simulink library "DSP_FPGA_Accelerated_Toolbox"  (R2019b)
settings: Solver=VariableStepAuto  StartTime=0.0  StopTime=10.0  RelTol=1e-3
undefined symbols (not defined in the file or in its folder): a, b, c
libraries: hdlsllib x72, simulink x19, $bdroot x2
(part 1 of 3)
settings Model: Creator=E. Bailey Galacci  LastModifiedBy=Balad
settings SFSimCC: CustomCodeUndefinedFunction=UseInterfaceOnly

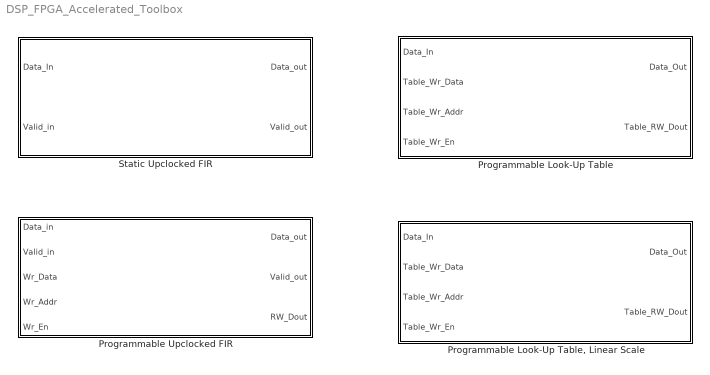
== system DSP_FPGA_Accelerated_Toolbox ==
  Programmable Look-Up Table : Subsystem  mask(Programmable Look-Up Table){TableFn=X_in.^0.5, maxInput=1, floor_in_tab=2^-15, error_cap_tab=.1, ERR_DIAG=off, N_bits_tab=4, M_bits_tab=5, igotthis=off, W_bits=32, F_bits=28, Table_Init=0, d=0}
      mask prompts: TableFn "Table Represented Function"; maxInput "Maximum Input Value"; floor_in_tab "Minimum Input Threshold"; error_cap_tab "Maximum Allowed Error (%)"; ERR_DIAG "Show Error Calculation"; N_bits_tab "N_bits"; M_bits_tab "M_bits"; igotthis "Manual Bit Definition Override"; W_bits "Word Bits"; F_bits "Fractional Bits"
      mask help:
      | A hardware-oriented implementation of a lookup table.
      | Provides a fairly resource efficient way to avoid hardware-difficult operations, such as logarithms or square roots.
      | Tables can be initialized on system startup and rewritten during runtime using the Table_Wr lines.
      | Min input cannot be 0, because inputs are pseudo-logarithmically spaced.
      mask init:
      | % things to display: table size, floor input?, max input, accuracy
      | % things to figure out: M_bits, N_bits, Min_val, X_in table, Y_out table,
      | % max_error, ram_size, table_size 
      | 
      | d = ceil(log2(maxInput));
      | if(igotthis)
      |     N_bits = N_bits_tab;
      |     M_bits = M_bits_tab;
      | else
      |     N_bits = ceil(log2(d-log2(floor_in_tab)+1));
      |     % M_bits needs to be defined later, as it must be just enough to meet
      |     % accuracy standards defined by user, with linear interpolation
      |     M_bits = 1; %this will be updated later as needed
      | end;
      | 
      | repeatFlag = true;
      | while(repeatFlag)
      |     % Define a N point log2 spaced range of inputs, from 2^(d-(2^N_bits -1)) to almost 2^(d+1), 
      |     % this effectively covers the user defined input range, down to a floor
      |     % value.
      |     X_in = zeros(1, 2^(M_bits+N_bits));
      |     addr = 1;
      |     for NShifts = 2^N_bits-1:-1:0
      |         for M = 0:2^M_bits - 1
      |             X_in(addr) = 2^(d-NShifts) + M*2^(d-NShifts-M_bits);
      |             addr = addr+1;
      |         end
      |     end
      | 
      |     % use function to define output. note: function must contain input X_in
      |     % within the string to work properly, and the only output of the function
      |     % must be Y_out.
      |     Y_out = eval(TableFn);
      | 
      |     ram_size = N_bits+M_bits;
      |     Table_Init = Y_out;
      |     figure(2); plot(X_in,Y_out, 'k*'); title('Table Initialized Function');
      |     max_val = 2^d+ (2^M_bits -1)*2^(d-M_bits);
      |     min_val = 2^(d-(2^N_bits-1));
      |     %set_param(gcb,'MaskDisplay',"disp(sprintf('Programmable Look-up Table\nMemory Used = %d samples and coeffs\nClock Rate Needed = %d Hz', FIR_Uprate*2, Max_Rate)); port_label('input',1,'data'); port_label('input',2,'valid'); port_label('input',3,'Wr_Data'); port_label('input',4,'Wr_Addr'); port_label('input',5,'Wr_En'); port_label('output',1,'data'); port_label('output',2,'valid'); port_label('output',3,'RW_Dout');")
      | 
      |     %%%%%%%%%% check and identify error %%%%%%%%%%%
      |     % Make some values for an "ideal" lookup table with log spaced points
      |     X_in_Ideal = logspace(log10(min_val), log10(max_val), 2^(ram_size+2));
      |     X_temp = X_in;
      |     X_in = X_in_Ideal;
      |     % identify the values of the function at X_in_Ideal
      |     Y_out_Ideal = eval(TableFn);
      | 
      |     % Get values for lookup table (already have X_in)
      |     X_in = X_temp;
      | 
      |     % Find lookup addresses for each point in X_in_Ideal
      |     x_addr = zeros(1,length(X_in_Ideal));
      |     for it = 1:length(X_in_Ideal)
      |         x_addr(it) = 2^ram_size;
      |         X_Shift = X_in_Ideal(it);
      |         while(X_Shift < X_in(x_addr(it)) && x_addr(it) ~= 1)
      |             x_addr(it) = x_addr(it) - 1;
      |         end
      |         if(x_addr(it)==0)
      |             x_addr(it) = 1;
      |         end
      |     end
      | 
      |     % Check for any possible out of bounds errors (handled similarly in
      |     % hardware)
      |     x_addr(x_addr == 2^ram_size) = 2^ram_size -1;
      | 
      |     % Get values for linear interpolation of X_in_Ideal
      |     x_low  = X_in(x_addr);
      |     x_high = X_in(x_addr+1);
      | 
      | 
      |     y_low  = Y_out(x_addr);
      |     y_high = Y_out(x_addr+1);
      |     slope  = (y_high-y_low) ./ (x_high - x_low);
      |     y_inter = slope.*(X_in_Ideal-x_low)+y_low;
      |     % percent error: obt-exp / exp
      |     %errorFloor = (Y_out_Ideal-y_low)./Y_out_Ideal;
      |     errorInter = (Y_out_Ideal-y_inter)./Y_out_Ideal;
      |     %maxFloorErr(ix) = 100*max(abs(errorFloor(ix, 2870:9839)));
      |     %maxInterErr(ix) = 100*max(abs(errorInter(ix, 2870:9839)));
      |     maxErr = max(abs(errorInter));
      |     
      |     %check while loop condition
      |     if(igotthis) 
      |         repeatFlag = false;
      |     else
      |         if(maxErr <= .01*error_cap_tab)
      |             repeatFlag = false;
      |             if(ERR_DIAG)
      |                 figure(1); 
      |                 subplot(2,1,1); semilogx(X_in_Ideal,y_inter, X_in_Ideal,Y_out_Ideal,X_in,Y_out,'k*'); title('Output Values over Input Range'); xlabel('Inputs'); ylabel('Outputs'); legend('Interpolated','Ideal','Table Points');
      |                 subplot(2,1,2); semilogx(X_in_Ideal,100*errorInter); title('Error of Output over Input Range'); xlabel('Inputs'); ylabel('Percent Error');
      |             end
      |         else
      |             if(ERR_DIAG)
      |                 f = msgbox(sprintf('Err = %.2d, M_bits = %d', maxErr, M_bits),'Configuring PLUT','replace');
      |             end
      |             if(maxErr > 8*.01*error_cap_tab)
      |                 M_bits = M_bits+3;
      |             elseif(maxErr > 4*.01*error_cap_tab)
      |                 M_bits = M_bits+2;
      |             else
      |                 M_bits = M_bits+1;
      |             end
      |         end
      |     end
      | end%end while loop
      | 
      | %maxFloorErrTot = max(maxFloorErr);
      | %maxInterErrTot = max(maxInterErr);
      | % things to display: table size, floor input?, max input, accuracy
      | 
      | set_param(gcb,'MaskDisplay',"disp(sprintf('Programmable Look-Up Table\nMemory Used = %d fixed point numbers\nInput Bounds: %.2d <= x <= %.2d\n Maximum Error: %.2d %', 2*2^ram_size, min_val, max_val, 100*maxErr)); port_label('input',1,'Data_In'); port_label('input',2,'Table_Wr_Data'); port_label('input',3,'Table_Wr_Addr'); port_label('input',4,'Table_Wr_En'); port_label('output',1,'Data_Out'); port_label('output',2,'Table_RW_Dout');")
      mask Help:
      | A hardware-oriented implementation of a lookup table.
      | Provides a fairly resource efficient way to avoid hardware-difficult operations, such as logarithms or square roots.
      | Tables can be initialized on system startup and rewritten during runtime using the Table_Wr lines.
      | Min input cannot be 0, because inputs are pseudo-logarithmically spaced.
      | 
      | Uses pseudo-logarithmic spacing of inputs for maximum accuracy in non-linear functions, as well as linear interpolation between points to further increase accuracy. Because of this, it is assumed that function input is unsigned. If this is undesired, a second table would need to be implemented to cover negative values, or some other solution outside the block.
      | 
      | Capable of automatically determining required table size to meet a given accuracy requirement within the entire data range, or can be manually set to a specific size with M_bits and N_bits. N_bits determines the data range as a power of 1/2 of the maximum input. M_bits determines the number of bits in the address used to increase function precision, by increasing the number of points stored between each log2 spaced input point.
      | 
      | 
      | 
      | ------------------
      | Mask Parameters
      | ------------------
      | 
      | Table Represented Function:
      |   Function to estimate using the lookup table. Must contain the variable "X_in" as an input to a function, or as a variable within the executable code string, as this is used in the Initialization code to evaluate the function. If a function, that function must also have a single output which will define the values to fill the table with given input value X_in.
      | 
      | --Table Parameters--
      |   Maximum Input Value:
      |     The maximum input value the table should be expected to represent. If the input value is greater than this parameter's nearest higher power of 2
      | 
      | ----------
      | Block I/O
      | ----------
      mask DialogControl Control2_copy Prompt: Must be a function of X_in to get Y_out
      mask DialogControl Container3 Prompt: Table Parameters
      mask DialogControl Container5 Prompt: Define Input Threshold and Accuracy
      mask DialogControl Container7 Prompt: Define Addresses Space Manually
      mask DialogControl Control2 Prompt: See Documentation for details
      mask DialogControl Container9 Prompt: Data Parameters (In Testing)
      mask Display: disp(sprintf('Programmable Look-Up Table\nMemory Used = %d fixed point numbers\nInput Bounds: %.2d <= x <= %.2d\n Maximum Error: %.2d %', 2*2^ram_size, min_val, max_val, 100*maxErr)); port_label('input',1,'Data_In'); port_label('input',2,'Table_Wr_Data'); port_label('input',3,'Table_Wr_Addr'); port_label('input',4,'Table_Wr_En'); port_label('output',1,'Data_Out'); port_label('output',2,'Table_RW_Dout');
  "Programmable Look-Up Table, Linear Scale" : Subsystem  mask(Programmable Look-Up Table){TableFn=X_in.^0.5, maxInput=1, floor_in_tab=2^-15, error_cap_tab=.1, ERR_DIAG=off, N_bits_tab=4, M_bits_tab=5, igotthis=off, W_bits=32, F_bits=28, Table_Init=0, d=0}
      mask prompts: TableFn "Table Represented Function"; maxInput "Maximum Input Value"; floor_in_tab "Minimum Input Threshold"; error_cap_tab "Maximum Allowed Error (%)"; ERR_DIAG "Show Error Calculation"; N_bits_tab "N_bits"; M_bits_tab "M_bits"; igotthis "Manual Bit Definition Override"; W_bits "Word Bits"; F_bits "Fractional Bits"
      mask help:
      | A hardware-oriented implementation of a lookup table.
      | Provides a fairly resource efficient way to avoid hardware-difficult operations, such as logarithms or square roots.
      | Tables can be initialized on system startup and rewritten during runtime using the Table_Wr lines.
      | Min input cannot be 0, because inputs are pseudo-logarithmically spaced.
      mask init: same as DSP_FPGA_Accelerated_Toolbox/Programmable Look-Up Table
      mask Help:
      | A hardware-oriented implementation of a lookup table.
      | Provides a fairly resource efficient way to avoid hardware-difficult operations, such as logarithms or square roots.
      | Tables can be initialized on system startup and rewritten during runtime using the Table_Wr lines.
      | Min input cannot be 0, because inputs are pseudo-logarithmically spaced.
      | 
      | Uses pseudo-logarithmic spacing of inputs for maximum accuracy in non-linear functions, as well as linear interpolation between points to further increase accuracy. Because of this, it is assumed that function input is unsigned. If this is undesired, a second table would need to be implemented to cover negative values, or some other solution outside the block.
      | 
      | Capable of automatically determining required table size to meet a given accuracy requirement within the entire data range, or can be manually set to a specific size with M_bits and N_bits. N_bits determines the data range as a power of 1/2 of the maximum input. M_bits determines the number of bits in the address used to increase function precision, by increasing the number of points stored between each log2 spaced input point.
      | 
      | 
      | 
      | ------------------
      | Mask Parameters
      | ------------------
      | 
      | Table Represented Function:
      |   Function to estimate using the lookup table. Must contain the variable "X_in" as an input to a function, or as a variable within the executable code string, as this is used in the Initialization code to evaluate the function. If a function, that function must also have a single output which will define the values to fill the table with given input value X_in.
      | 
      | --Table Parameters--
      |   Maximum Input Value:
      |     The maximum input value the table should be expected to represent. If the input value is greater than this parameter's nearest higher power of 2
      | 
      | ----------
      | Block I/O
      | ----------
      mask DialogControl Control2_copy Prompt: Must be a function of X_in to get Y_out
      mask DialogControl Container3 Prompt: Table Parameters
      mask DialogControl Container5 Prompt: Define Input Threshold and Accuracy
      mask DialogControl Container7 Prompt: Define Addresses Space Manually
      mask DialogControl Control2 Prompt: See Documentation for details
      mask DialogControl Container9 Prompt: Data Parameters (In Testing)
      mask Display: disp(sprintf('Programmable Look-Up Table\nMemory Used = %d fixed point numbers\nInput Bounds: %.2d <= x <= %.2d\n Maximum Error: %.2d %', 2*2^ram_size, min_val, max_val, 100*maxErr)); port_label('input',1,'Data_In'); port_label('input',2,'Table_Wr_Data'); port_label('input',3,'Table_Wr_Addr'); port_label('input',4,'Table_Wr_En'); port_label('output',1,'Data_Out'); port_label('output',2,'Table_RW_Dout');
  Programmable Upclocked FIR : Subsystem  mask(Programmable Upclocked FIR){B_k=[0.5,0.5], Ts=1/48000, Ts_system=1/98000, Added_Delay=0, W_bits=32, F_bits=28, Max_Rate=48000}
      mask prompts: B_k "B_k coefficients (vector)"; Ts "Sample Rate"; Ts_system "System Rate"; Added_Delay "Added Delay"; W_bits "Fixed Point Word Size"; F_bits "Fixed Point Frac Size"
      mask help:
      | This block is designed for a hardware implementation of an FIR filter. The main advantage is resource sharing by using a single multiply/add at an increased clock rate to multiply the b_k coefficients and sum the results.
      | The cost is a slightly increased amount of RAM used and the requirement that the system can run at data_rate*b_k_length, where b_k_length is rounded up to the nearest power of 2. The gains over a traditional FIR are a vastly decreased latency and logic resource usage.
      mask init:
      | FIR_Size = ceil(log2(length(B_k+Added_Delay)));
      | FIR_Uprate = 2^FIR_Size;
      | B_k_init = zeros(1,FIR_Uprate);
      | B_k_init(1:length(B_k)) = B_k;
      | Max_Rate = 1/(Ts/FIR_Uprate);
      | 
      | set_param(gcb,'MaskDisplay',"disp(sprintf('Programmable Clock-Accelerated FIR\nMemory Used = %d samples and coeffs\nClock Rate Needed = %d Hz', FIR_Uprate*2, Max_Rate)); port_label('input',1,'data'); port_label('input',2,'valid'); port_label('input',3,'Wr_Data'); port_label('input',4,'Wr_Addr'); port_label('input',5,'Wr_En'); port_label('output',1,'data'); port_label('output',2,'valid'); port_label('output',3,'RW_Dout');")
      mask Help:
      | This block is designed for a hardware implementation of an FIR filter. The main advantage is resource sharing by using a single multiply/add at an increased clock rate to multiply the b_k coefficients and sum the results.
      | The cost is a slightly increased amount of RAM used and the requirement that the system can run at data_rate*b_k_length, where b_k_length is rounded up to the nearest power of 2. The gains over a traditional FIR are a vastly decreased latency and logic resource usage.
      | 
      | An "Added Delay" option is included as a way to save resources when delaying the filtered signal. The b_k RAM is padded with 0s to round length up to a power of 2. Therefore, many faster cycles are completely uneccessary. Since many b_k's are 0, they can be rotated to align with inputs starting before the most recent, effectively delaying the output signal with 0 extra resources used. Useful for things like realigning a signal after multi-channel processing, or any other reason to delay the signal. If Added Delay would cause rotation to read from undesired coefficients (not 0), on startup the system will automatically increase the size of the table. This doubles the RAM used, so if using a b_k length at or near a power of 2, or if a very long delay is required, this may not be the most efficient option.
      | 
      | B_k's are defined on system start-up and can be changed during runtime through the Wr_Data, Wr_Addr, and Wr_En signals.
      | B_k's can be ready using the Wr_Addr, Wr_En set to 0, sent out to the RW_Dout line.
      | 
      | ------------------
      | Mask Parameters
      | ------------------
      | 
      | B_k coefficients:
      |   FIR filter coefficients
      | Sample Time:
      |   Amount of time between valid pulses, when the input signal needs to be recognized.
      | System Time:
      |   Amount of time between system clock cycles. Can be the same as Sample Time if Valid_in is always 1.
      | Added Delay:
      |   Adds a N-sample delay to the output. Check Documentation Description for details.
      | Fixed Point Word/Frac Size:
      |   Word and Fractional bit size of input and table data type. Data input and b_k's are assumed to be the same data type.
      | 
      | ----------
      | Block I/O
      | ----------
      | 
      | Data_in:
      |   Input signal to be processed. Can be of any rate a direct multiple of "Sample rate". Signed Fixed Point of size "Fixed Point Word Size".
      | Valid_in:
      |  Trigger to show input signal should be written to signal memory of FIR RAM. Active high. Boolean.
      | Wr_Data:
      |   Data to write to B_k at address Wr_Addr if Wr_En is set to 1. Data type overwritten to match input signal type.
      | Wr_Addr:
      |   Location in table to write or read B_k table. Starts at 0 and ends at 2^N, where N is ceil(log2(length(B_k+Added_Delay)));
      | Wr_En:
      |   Used to set behavior to read or write from b_k memory.
      |   Write: 1, Read: 0
      | 
      | Data_out:
      |   Output signal after processing. Set to sample time "System Time". Signed Fixed Point of size "Fixed Point Word Size". Zero-order hold.
      | Valid_out:
      |   Signal identifying when the output is a new processed value. Active high. Boolean.
      | RW_Dout:
      |   Returns the value stored in Wr_Addr, after a 1 System clock cycle delay.
      mask Display: disp(sprintf('Programmable Clock-Accelerated FIR\nMemory Used = %d samples and coeffs\nClock Rate Needed = %d Hz', FIR_Uprate*2, Max_Rate)); port_label('input',1,'data'); port_label('input',2,'valid'); port_label('input',3,'Wr_Data'); port_label('input',4,'Wr_Addr'); port_label('input',5,'Wr_En'); port_label('output',1,'data'); port_label('output',2,'valid'); port_label('output',3,'RW_Dout');
  Static Upclocked FIR : Subsystem  mask(Static Upclocked FIR){B_k=[0.5,0.5], Ts=1/48000, Ts_system=1/96000, Added_Delay=0, W_bits=32, F_bits=28, Max_Rate=48000}
      mask prompts: B_k "B_k coefficients (vector)"; Ts "Sample Time"; Ts_system "System Time"; Added_Delay "Added Delay"; W_bits "Fixed Point Word Size"; F_bits "Fixed Point Frac Size"
      mask help:
      | This block is designed for a hardware implementation of an FIR filter. The main advantage is resource sharing by using a single multiply/add at an increased clock rate to multiply the b_k coefficients and sum the results.
      | The cost is a slightly increased amount of RAM used and the requirement that the system can run at data_rate*b_k_length, where b_k_length is rounded up to the nearest power of 2. The gains over a traditional FIR are a vastly decreased latency and logic resource usage.
      mask init:
      | FIR_Size = ceil(log2(length(B_k+Added_Delay)));
      | FIR_Uprate = 2^FIR_Size;
      | B_k_init = zeros(1,FIR_Uprate);
      | B_k_init(1:length(B_k)) = B_k;
      | Max_Rate = 1/(Ts/FIR_Uprate);
      | 
      | set_param(gcb,'MaskDisplay',"disp(sprintf('Static Clock-Accelerated FIR\nMemory Used = %d samples and coeffs\nClock Rate Needed = %d Hz', FIR_Uprate*2, Max_Rate)); port_label('input',1,'data'); port_label('input',2,'valid'); port_label('output',1,'data'); port_label('output',2,'valid');")
      mask Help:
      | This block is designed for a hardware implementation of an FIR filter. The main advantage is resource sharing by using a single multiply/add at an increased clock rate to multiply the b_k coefficients and sum the results.
      | The cost is a slightly increased amount of RAM used and the requirement that the system can run at data_rate*b_k_length, where b_k_length is rounded up to the nearest power of 2. The gains over a traditional FIR are a vastly decreased latency and logic resource usage.
      | 
      | An "Added Delay" option is included as a way to save resources when delaying the filtered signal. The b_k RAM is padded with 0s to round length up to a power of 2. Therefore, many faster cycles are completely uneccessary. Since many b_k's are 0, they can be rotated to align with inputs starting before the most recent, effectively delaying the output signal with 0 extra resources used. Useful for things like realigning a signal after multi-channel processing, or any other reason to delay the signal. If Added Delay would cause rotation to read from undesired coefficients (not 0), on startup the system will automatically increase the size of the table. This doubles the RAM used, so if using a b_k length at or near a power of 2, or if a very long delay is required, this may not be the most efficient option.
      | 
      | 
      | B_k's are defined on system start-up and cannot be changed during runtime.
      | 
      | ------------------
      | Mask Parameters
      | ------------------
      | 
      | B_k coefficients:
      |   FIR filter coefficients
      | Sample Time:
      |   Amount of time between valid pulses, when the input signal needs to be recognized.
      | System Time:
      |   Amount of time between system clock cycles. Can be the same as Sample Time if Valid_in is always 1.
      | Added Delay:
      |   Adds a N-sample delay to the output. Check Documentation Description for details.
      | Fixed Point Word/Frac Size:
      |   Word and Fractional bit size of input and table data type. Data input and b_k's are assumed to be the same data type.
      | 
      | ----------
      | Block I/O
      | ----------
      | 
      | Data_in:
      |   Input signal to be processed. Can be of any rate a direct multiple of "Sample rate". Signed Fixed Point of size "Fixed Point Word Size".
      | Valid_in:
      |  Trigger to show input signal should be written to signal memory of FIR RAM. Active high. Boolean.
      | 
      | Data_out:
      |   Output signal after processing. Set to sample time "System Time". Signed Fixed Point of size "Fixed Point Word Size". Zero-order hold.
      | Valid_out:
      |   Signal identifying when the output is a new processed value. Active high. Boolean.
      mask DialogControl B_k Tooltip: Filter Coefficients
      mask DialogControl Ts Tooltip: Ts
      mask DialogControl Ts_system Tooltip: Ts_system
      mask DialogControl Added_Delay Tooltip: An efficient way to realign signals
      mask DialogControl W_bits Tooltip: W_bits, size of Fixed Point word
      mask DialogControl F_bits Tooltip: F_bits, size of fractional component of word
      mask Display: disp(sprintf('Static Clock-Accelerated FIR\nMemory Used = %d samples and coeffs\nClock Rate Needed = %d Hz', FIR_Uprate*2, Max_Rate)); port_label('input',1,'data'); port_label('input',2,'valid'); port_label('output',1,'data'); port_label('output',2,'valid');

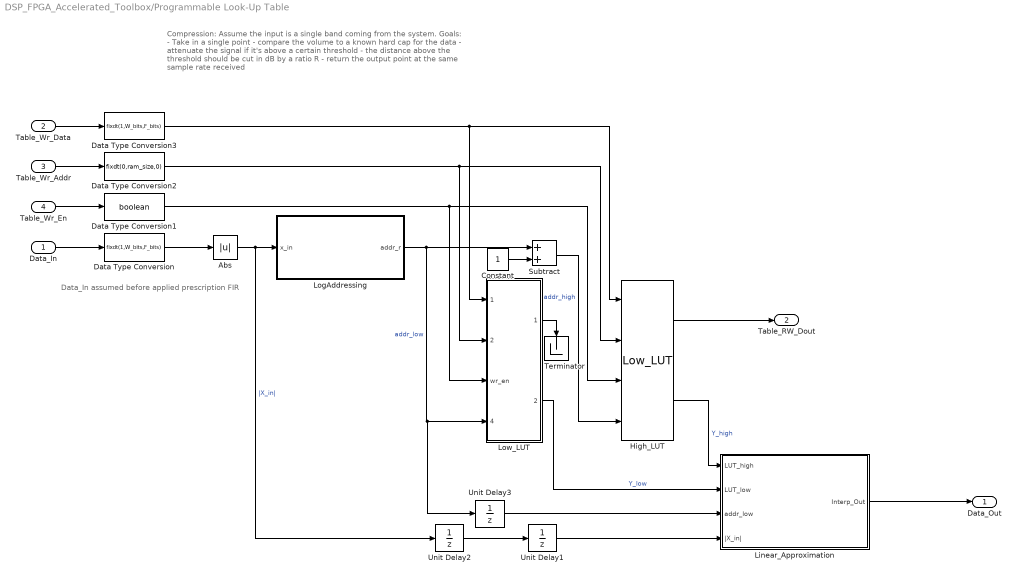
== system DSP_FPGA_Accelerated_Toolbox/Programmable Look-Up Table ==
  note: Data_In assumed before applied prescription FIR
  note: Compression: Assume the input is a single band coming from the system.
      |
      | Goals:
      | 	- Take in a single point
      | 	- compare the volume to a known hard cap for the data
      | 	- attenuate the signal if it's above a certain threshold
      | 		- the distance above the threshold should be cut in dB by a ratio R
      | 	- return the output point at the same sample rate received
  Data_In : Inport
  Table_Wr_Data : Inport  Port=2
  Table_Wr_Addr : Inport  Port=3
  Table_Wr_En : Inport  Port=4
  Abs : Abs
  Constant : Constant  OutDataTypeStr=fixdt(0,ram_size,0)  SampleTime=-1
  Data Type Conversion : DataTypeConversion  OutDataTypeStr=fixdt(1,W_bits,F_bits)
  Data Type Conversion1 : DataTypeConversion  OutDataTypeStr=boolean
  Data Type Conversion2 : DataTypeConversion  OutDataTypeStr=fixdt(0,ram_size,0)
  Data Type Conversion3 : DataTypeConversion  OutDataTypeStr=fixdt(1,W_bits,F_bits)
  High_LUT : $bdroot/Programmable Look-Up Table/Low_LUT  ram_size=N_bits+M_bits  Table_Init=Table_Init
  Linear_Approximation : Subsystem
  LogAddressing : Subsystem
  Low_LUT : Subsystem  mask(Dual-port RAM){ram_size=N_bits+M_bits, Table_Init=Table_Init}
      mask prompts: ram_size "Address port width (2 to 29 bits)"; Table_Init "Table Initialized Values"
      mask help: This block simulates a dual-port RAM with two data output ports.
      mask init:
      | hdlblkmask_dpram;
      mask Help: helpview([docroot '/simulink/helptargets.map'],'HDL_dual_port_RAM');
  Subtract : Sum  OutDataTypeStr=Inherit: Same as first input
  Terminator : Terminator
  Unit Delay1 : UnitDelay  InitialCondition=1  SampleTime=-1  HasFrameUpgradeWarning=on
  Unit Delay2 : UnitDelay  InitialCondition=1  SampleTime=-1  HasFrameUpgradeWarning=on
  Unit Delay3 : UnitDelay  InitialCondition=1  SampleTime=-1  HasFrameUpgradeWarning=on
  Data_Out : Outport  VectorParamsAs1DForOutWhenUnconnected=off
  Table_RW_Dout : Outport  Port=2  VectorParamsAs1DForOutWhenUnconnected=off
  wires:
  Table_Wr_Data/1 -> Data Type Conversion3/1
  Table_Wr_En/1 -> Data Type Conversion1/1
  Table_Wr_Addr/1 -> Data Type Conversion2/1
  LogAddressing/1(addr_r) -> Low_LUT/4(rd_addr), Unit Delay3/1, Subtract/1  "addr_low"
  Abs/1 -> Unit Delay2/1, LogAddressing/1(x_in)  "|X_in|"
  Data_In/1 -> Data Type Conversion/1
  Constant/1 -> Subtract/2
  Subtract/1 -> High_LUT/4  "addr_high"
  Low_LUT/1(wr_dout) -> Terminator/1
  High_LUT/1 -> Table_RW_Dout/1
  High_LUT/2 -> Linear_Approximation/1(LUT_high)  "Y_high"
  Low_LUT/2(rd_dout) -> Linear_Approximation/2(LUT_low)  "Y_low"
  Linear_Approximation/1(Interp_Out) -> Data_Out/1
  Unit Delay2/1 -> Unit Delay1/1
  Unit Delay1/1 -> Linear_Approximation/4(|X_in|)
  Unit Delay3/1 -> Linear_Approximation/3(addr_low)
  Data Type Conversion/1 -> Abs/1
  Data Type Conversion1/1 -> High_LUT/3, Low_LUT/3(wr_en)
  Data Type Conversion2/1 -> High_LUT/2, Low_LUT/2(wr_addr)
  Data Type Conversion3/1 -> High_LUT/1, Low_LUT/1(wr_din)

== system DSP_FPGA_Accelerated_Toolbox/Programmable Look-Up Table, Linear Scale ==
  note: Data_In assumed before applied prescription FIR
  note: Compression: Assume the input is a single band coming from the system.
      |
      | Goals:
      | 	- Take in a single point
      | 	- compare the volume to a known hard cap for the data
      | 	- attenuate the signal if it's above a certain threshold
      | 		- the distance above the threshold should be cut in dB by a ratio R
      | 	- return the output point at the same sample rate received
  Data_In : Inport
  Table_Wr_Data : Inport  Port=2
  Table_Wr_Addr : Inport  Port=3
  Table_Wr_En : Inport  Port=4
  Data Type Conversion : DataTypeConversion  OutDataTypeStr=fixdt(1,W_bits,F_bits)
  Data Type Conversion1 : DataTypeConversion  OutDataTypeStr=boolean
  Data Type Conversion2 : DataTypeConversion  OutDataTypeStr=fixdt(0,ram_size,0)
  Data Type Conversion3 : DataTypeConversion  OutDataTypeStr=fixdt(1,W_bits,F_bits)
  LinAddressing : Subsystem
  Low_LUT : Subsystem  mask(Dual-port RAM){ram_size=N_bits+M_bits, Table_Init=Table_Init}
      mask prompts: ram_size "Address port width (2 to 29 bits)"; Table_Init "Table Initialized Values"
      mask help: This block simulates a dual-port RAM with two data output ports.
      mask init:
      | hdlblkmask_dpram;
      mask Help: helpview([docroot '/simulink/helptargets.map'],'HDL_dual_port_RAM');
  Data_Out : Outport  VectorParamsAs1DForOutWhenUnconnected=off
  Table_RW_Dout : Outport  Port=2  VectorParamsAs1DForOutWhenUnconnected=off
  wires:
  Table_Wr_Data/1 -> Data Type Conversion3/1
  Table_Wr_En/1 -> Data Type Conversion1/1
  Table_Wr_Addr/1 -> Data Type Conversion2/1
  LinAddressing/1(addr_r) -> Low_LUT/4(rd_addr)  "addr"
  Data Type Conversion/1 -> LinAddressing/1(x_in)  "x_in"
  Data_In/1 -> Data Type Conversion/1
  Low_LUT/1(wr_dout) -> Table_RW_Dout/1
  Data Type Conversion1/1 -> Low_LUT/3(wr_en)
  Data Type Conversion2/1 -> Low_LUT/2(wr_addr)
  Data Type Conversion3/1 -> Low_LUT/1(wr_din)
  Low_LUT/2(rd_dout) -> Data_Out/1  "Y_low"

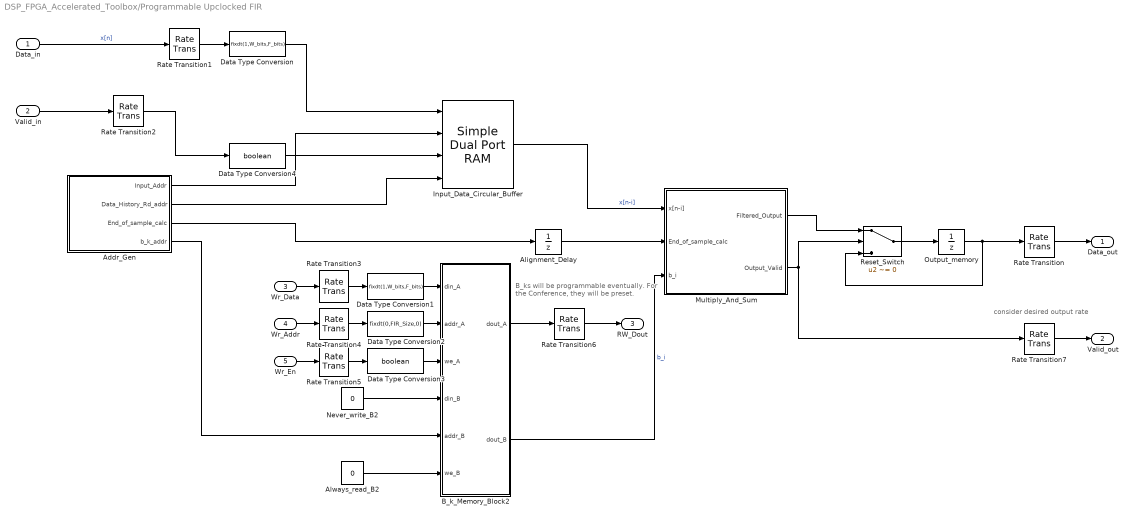
== system DSP_FPGA_Accelerated_Toolbox/Programmable Upclocked FIR ==
  note: consider desired output rate
  note: B_ks will be programmable eventually.
      | For the Conference, they will be preset.
  Data_in : Inport
  Valid_in : Inport  Port=2
  Wr_Data : Inport  Port=3
  Wr_Addr : Inport  Port=4
  Wr_En : Inport  Port=5
  "Addr_Gen " : Subsystem
  Alignment_Delay : UnitDelay  SampleTime=-1  HasFrameUpgradeWarning=on
  Always_read_B2 : Constant  Value=0  OutDataTypeStr=boolean  SampleTime=Ts/FIR_Uprate
  B_k_Memory_Block2 : Subsystem  mask(Dual-rate dual-port RAM){ram_size=FIR_Size, B_k_init=B_k_init}
      mask prompts: ram_size "Address port width (2 to 28 bits)"
      mask help: This block simulates a dual-clock dual-port RAM with two data output ports.
      mask init:
      | hdlblkmask_drdpram();
      mask Help: helpview([docroot '/simulink/helptargets.map'],'HDL_dual_rate_dual_port_ram');
  Data Type Conversion : DataTypeConversion  OutDataTypeStr=fixdt(1,W_bits,F_bits)
  Data Type Conversion1 : DataTypeConversion  OutDataTypeStr=fixdt(1,W_bits,F_bits)
  Data Type Conversion2 : DataTypeConversion  OutDataTypeStr=fixdt(0,FIR_Size,0)
  Data Type Conversion3 : DataTypeConversion  OutDataTypeStr=boolean
  Data Type Conversion4 : DataTypeConversion  OutDataTypeStr=boolean
  Input_Data_Circular_Buffer : hdlsllib/HDL RAMs/Simple Dual Port RAM  ram_size=FIR_Size
      settings: SourceProductName=Simulink  SourceProductBaseCode=SL
  Multiply_And_Sum : Subsystem
  Never_write_B2 : Constant  Value=0  OutDataTypeStr=fixdt(1, W_bits, F_bits)  SampleTime=Ts/FIR_Uprate
  Output_memory : UnitDelay  SampleTime=-1  HasFrameUpgradeWarning=on
  Rate Transition : RateTransition  OutPortSampleTime=Ts_system
  Rate Transition{1..5} (5 alike) : RateTransition  OutPortSampleTime=Ts/FIR_Uprate
  Rate Transition6 : RateTransition  OutPortSampleTime=Ts_system
  Rate Transition7 : RateTransition  OutPortSampleTime=Ts_system
  Reset_Switch : Switch  Criteria=u2 ~= 0
  Data_out : Outport  VectorParamsAs1DForOutWhenUnconnected=off
  Valid_out : Outport  Port=2  VectorParamsAs1DForOutWhenUnconnected=off
  RW_Dout : Outport  Port=3  VectorParamsAs1DForOutWhenUnconnected=off
  wires:
  Rate Transition2/1 -> Data Type Conversion4/1
  Rate Transition1/1 -> Data Type Conversion/1
  Alignment_Delay/1 -> Multiply_And_Sum/2(End_of_sample_calc)
  "Addr_Gen "/4(b_k_addr) -> B_k_Memory_Block2/5(addr_B)
  Output_memory/1 -> Rate Transition/1, Reset_Switch/3
  Valid_in/1 -> Rate Transition2/1
  Never_write_B2/1 -> B_k_Memory_Block2/4(din_B)
  Multiply_And_Sum/1(Filtered_Output) -> Reset_Switch/1
  Data_in/1 -> Rate Transition1/1  "x[n]"
  "Addr_Gen "/3(End_of_sample_calc) -> Alignment_Delay/1
  B_k_Memory_Block2/2(dout_B) -> Multiply_And_Sum/3(b_i)  "b_i"
  "Addr_Gen "/1(Input_Addr) -> Input_Data_Circular_Buffer/2
  Reset_Switch/1 -> Output_memory/1
  "Addr_Gen "/2(Data_History_Rd_addr) -> Input_Data_Circular_Buffer/4
  Rate Transition4/1 -> Data Type Conversion2/1
  Input_Data_Circular_Buffer/1 -> Multiply_And_Sum/1(x[n-i])  "x[n-i]"
  Rate Transition3/1 -> Data Type Conversion1/1
  Multiply_And_Sum/2(Output_Valid) -> Rate Transition7/1, Reset_Switch/2
  Always_read_B2/1 -> B_k_Memory_Block2/6(we_B)
  Rate Transition/1 -> Data_out/1
  Wr_Data/1 -> Rate Transition3/1
  Wr_Addr/1 -> Rate Transition4/1
  Rate Transition5/1 -> Data Type Conversion3/1
  Wr_En/1 -> Rate Transition5/1
  B_k_Memory_Block2/1(dout_A) -> Rate Transition6/1
  Rate Transition6/1 -> RW_Dout/1
  Rate Transition7/1 -> Valid_out/1
  Data Type Conversion/1 -> Input_Data_Circular_Buffer/1
  Data Type Conversion1/1 -> B_k_Memory_Block2/1(din_A)
  Data Type Conversion2/1 -> B_k_Memory_Block2/2(addr_A)
  Data Type Conversion3/1 -> B_k_Memory_Block2/3(we_A)
  Data Type Conversion4/1 -> Input_Data_Circular_Buffer/3

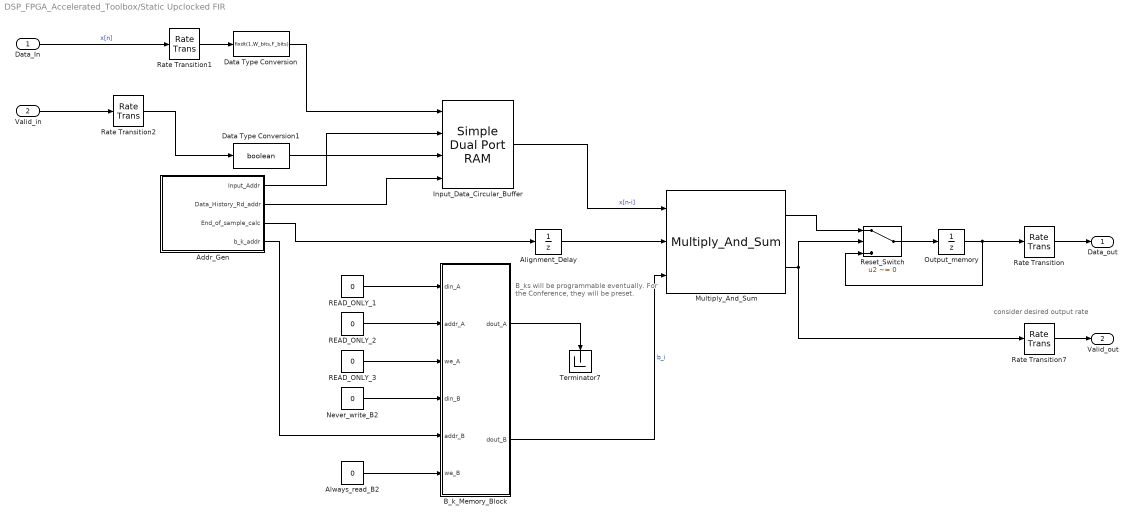
== system DSP_FPGA_Accelerated_Toolbox/Static Upclocked FIR ==
  note: consider desired output rate
  note: B_ks will be programmable eventually.
      | For the Conference, they will be preset.
  Data_In : Inport
  Valid_in : Inport  Port=2
  "Addr_Gen " : Subsystem
  Alignment_Delay : UnitDelay  SampleTime=-1  HasFrameUpgradeWarning=on
  Always_read_B2 : Constant  Value=0  OutDataTypeStr=boolean  SampleTime=Ts/FIR_Uprate
  B_k_Memory_Block : Subsystem  mask(Dual-rate dual-port RAM){ram_size=FIR_Size, B_k_init=B_k_init}
      mask prompts: ram_size "Address port width (2 to 28 bits)"
      mask help: This block simulates a dual-clock dual-port RAM with two data output ports.
      mask init:
      | hdlblkmask_drdpram();
      mask Help: helpview([docroot '/simulink/helptargets.map'],'HDL_dual_rate_dual_port_ram');
  Data Type Conversion : DataTypeConversion  OutDataTypeStr=fixdt(1,W_bits,F_bits)
  Data Type Conversion1 : DataTypeConversion  OutDataTypeStr=boolean
  Input_Data_Circular_Buffer : hdlsllib/HDL RAMs/Simple Dual Port RAM  ram_size=FIR_Size
      settings: SourceProductName=Simulink  SourceProductBaseCode=SL
  Multiply_And_Sum : $bdroot/Programmable Upclocked FIR/Multiply_And_Sum  SystemSampleTime=-1  Latency=0  AutoFrameSizeCalculation=off
  Never_write_B2 : Constant  Value=0  OutDataTypeStr=fixdt(1, W_bits, F_bits)  SampleTime=Ts/FIR_Uprate
  Output_memory : UnitDelay  SampleTime=-1  HasFrameUpgradeWarning=on
  READ_ONLY_1 : Constant  Value=0  OutDataTypeStr=fixdt(1, W_bits, F_bits)  SampleTime=Ts/FIR_Uprate
  READ_ONLY_2 : Constant  Value=0  OutDataTypeStr=fixdt(0,FIR_Size, 0)  SampleTime=Ts/FIR_Uprate
  READ_ONLY_3 : Constant  Value=0  OutDataTypeStr=boolean  SampleTime=Ts/FIR_Uprate
  Rate Transition : RateTransition  OutPortSampleTime=Ts_system
  Rate Transition1 : RateTransition  OutPortSampleTime=Ts/FIR_Uprate
  Rate Transition2 : RateTransition  OutPortSampleTime=Ts/FIR_Uprate
  Rate Transition7 : RateTransition  OutPortSampleTime=Ts_system
  Reset_Switch : Switch  Criteria=u2 ~= 0
  Terminator7 : Terminator
  Data_out : Outport  VectorParamsAs1DForOutWhenUnconnected=off
  Valid_out : Outport  Port=2  VectorParamsAs1DForOutWhenUnconnected=off
  wires:
  Rate Transition2/1 -> Data Type Conversion1/1
  Rate Transition1/1 -> Data Type Conversion/1
  Alignment_Delay/1 -> Multiply_And_Sum/2
  "Addr_Gen "/4(b_k_addr) -> B_k_Memory_Block/5(addr_B)
  Output_memory/1 -> Rate Transition/1, Reset_Switch/3
  Valid_in/1 -> Rate Transition2/1
  Never_write_B2/1 -> B_k_Memory_Block/4(din_B)
  READ_ONLY_3/1 -> B_k_Memory_Block/3(we_A)
  Multiply_And_Sum/1 -> Reset_Switch/1
  Data_In/1 -> Rate Transition1/1  "x[n]"
  "Addr_Gen "/3(End_of_sample_calc) -> Alignment_Delay/1
  B_k_Memory_Block/2(dout_B) -> Multiply_And_Sum/3  "b_i"
  "Addr_Gen "/1(Input_Addr) -> Input_Data_Circular_Buffer/2
  Reset_Switch/1 -> Output_memory/1
  "Addr_Gen "/2(Data_History_Rd_addr) -> Input_Data_Circular_Buffer/4
  READ_ONLY_2/1 -> B_k_Memory_Block/2(addr_A)
  Input_Data_Circular_Buffer/1 -> Multiply_And_Sum/1  "x[n-i]"
  READ_ONLY_1/1 -> B_k_Memory_Block/1(din_A)
  Multiply_And_Sum/2 -> Rate Transition7/1, Reset_Switch/2
  B_k_Memory_Block/1(dout_A) -> Terminator7/1
  Always_read_B2/1 -> B_k_Memory_Block/6(we_B)
  Rate Transition/1 -> Data_out/1
  Rate Transition7/1 -> Valid_out/1
  Data Type Conversion/1 -> Input_Data_Circular_Buffer/1
  Data Type Conversion1/1 -> Input_Data_Circular_Buffer/3

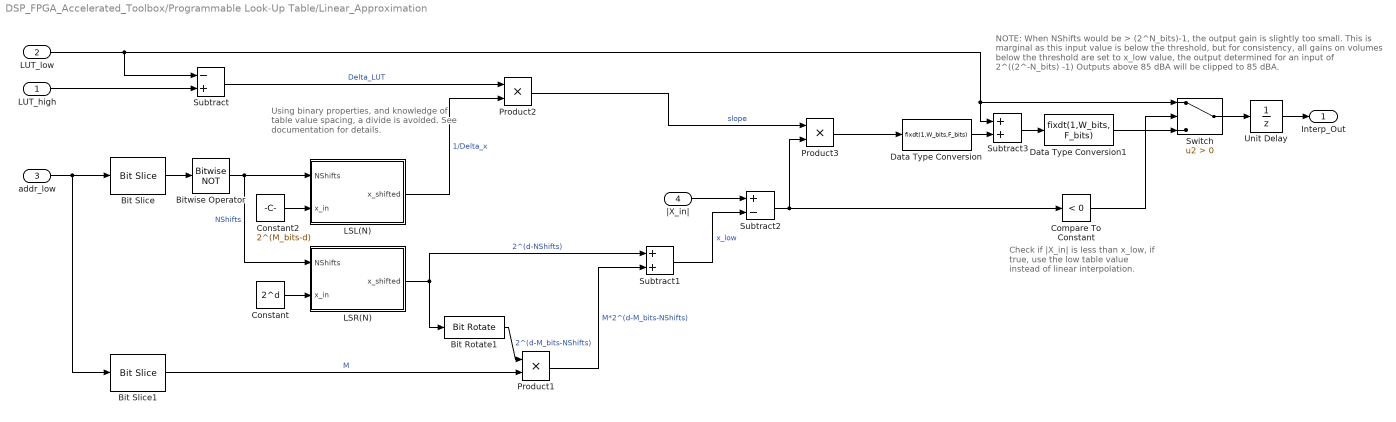
== system DSP_FPGA_Accelerated_Toolbox/Programmable Look-Up Table/Linear_Approximation ==
  note: Using binary properties, and knowledge
      | of table value spacing, a divide is avoided.
      | See documentation for details.
  note: Check if |X_in| is less than x_low,
      | if true, use the low table value
      | instead of linear interpolation.
  note: NOTE: When NShifts would be > (2^N_bits)-1, the output gain is slightly too small.
      | This is marginal as this input value is below the threshold, but for consistency,
      | all gains on volumes below the threshold are set to x_low value, the output determined
      | for an input of 2^((2^-N_bits)  -1)
      | Outputs above 85 dBA will be clipped to 85 dBA.
  LUT_high : Inport
  LUT_low : Inport  Port=2
  addr_low : Inport  Port=3
  |X_in| : Inport  Port=4
  Bit Rotate1 : hdlsllib/Logic and Bit Operations/Bit Rotate  mode=Rotate Right  N=M_bits
      settings: SourceProductName=Simulink  SourceProductBaseCode=SL
  Bit Slice : hdlsllib/Logic and Bit Operations/Bit Slice  lidx=M_bits+N_bits-1  ridx=M_bits
      settings: SourceProductName=Simulink  SourceProductBaseCode=SL
  Bit Slice1 : hdlsllib/Logic and Bit Operations/Bit Slice  lidx=M_bits-1  ridx=0
      settings: SourceProductName=Simulink  SourceProductBaseCode=SL
  Bitwise Operator : simulink/Logic and Bit Operations/Bitwise Operator  logicop=NOT  UseBitMask=off  BitMask=bin2dec('11011001')  BitMaskRealWorld=Stored Integer
  Compare To Constant : simulink/Logic and Bit Operations/Compare To Constant  relop=<  const=0  OutDataTypeStr=boolean
  Constant : Constant  Value=2^d  OutDataTypeStr=fixdt(0,W_bits,W_bits-2)  SampleTime=-1
  Constant2 : Constant  Value=2^(M_bits-d)  OutDataTypeStr=fixdt(0,W_bits,0)  SampleTime=-1
  Data Type Conversion : DataTypeConversion  OutDataTypeStr=fixdt(1,W_bits,F_bits)
  Data Type Conversion1 : DataTypeConversion  OutDataTypeStr=fixdt(1,W_bits, F_bits)
  LSL(N) : Subsystem
  LSR(N) : Subsystem
  Product1 : Product
  Product2 : Product
  Product3 : Product
  Subtract : Sum  Inputs=-+  OutDataTypeStr=Inherit: Same as first input
  Subtract1 : Sum  OutDataTypeStr=fixdt(1,W_bits, F_bits)
  Subtract2 : Sum  Inputs=+-  OutDataTypeStr=Inherit: Same as first input
  Subtract3 : Sum
  Switch : Switch  Criteria=u2 > Threshold
  Unit Delay : UnitDelay  InitialCondition=1  SampleTime=-1  HasFrameUpgradeWarning=on
  Interp_Out : Outport  VectorParamsAs1DForOutWhenUnconnected=off
  wires:
  addr_low/1 -> Bit Slice1/1, Bit Slice/1
  Bit Slice/1 -> Bitwise Operator/1
  Bitwise Operator/1 -> LSR(N)/1(NShifts), LSL(N)/1(NShifts)  "NShifts"
  Bit Slice1/1 -> Product1/2  "M"
  LUT_high/1 -> Subtract/2
  LUT_low/1 -> Subtract/1, Switch/1, Subtract3/1
  Subtract/1 -> Product2/1  "Delta_LUT"
  Constant/1 -> LSR(N)/2(x_in)
  LSR(N)/1(x_shifted) -> Subtract1/1, Bit Rotate1/1  "2^(d-NShifts)"
  Bit Rotate1/1 -> Product1/1  "2^(d-M_bits-NShifts)"
  Product1/1 -> Subtract1/2  "M*2^(d-M_bits-NShifts)"
  Subtract1/1 -> Subtract2/2  "x_low"
  LSL(N)/1(x_shifted) -> Product2/2  "1/Delta_x"
  Product2/1 -> Product3/1  "slope"
  |X_in|/1 -> Subtract2/1
  Subtract2/1 -> Compare To Constant/1, Product3/2
  Product3/1 -> Data Type Conversion/1
  Subtract3/1 -> Data Type Conversion1/1
  Constant2/1 -> LSL(N)/2(x_in)
  Data Type Conversion/1 -> Subtract3/2
  Data Type Conversion1/1 -> Switch/3
  Unit Delay/1 -> Interp_Out/1
  Compare To Constant/1 -> Switch/2
  Switch/1 -> Unit Delay/1

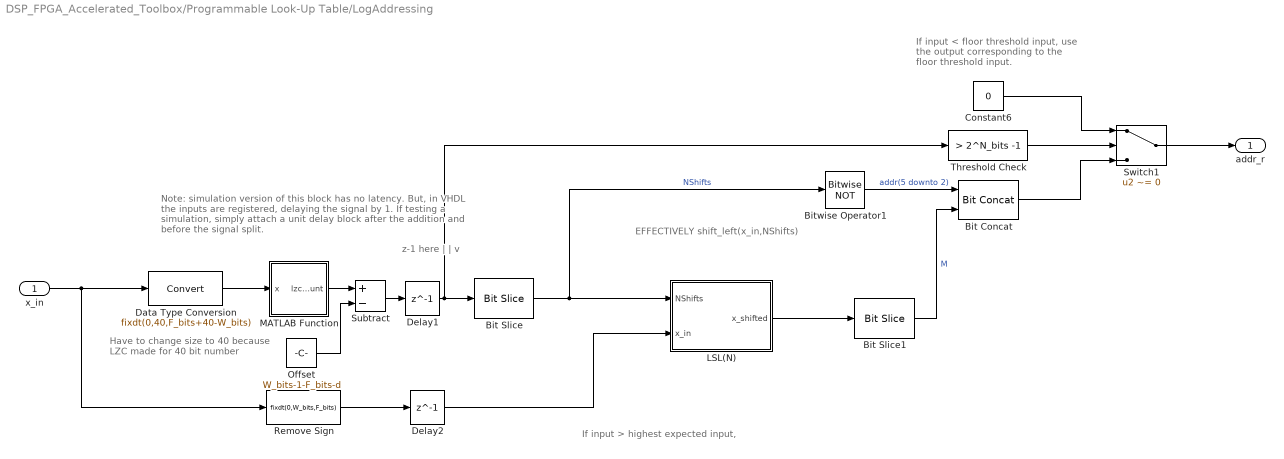
== system DSP_FPGA_Accelerated_Toolbox/Programmable Look-Up Table/LogAddressing ==
  note: z-1 here
      |    	|
      |    	|
      |   	v
  note: If input > highest expected input,
  note: If input < floor threshold input,
      | use the output corresponding to
      | the floor threshold input.
  note: Note: simulation version of this block has no latency.
      | But, in VHDL the inputs are registered, delaying the signal by 1.
      | If testing a simulation, simply attach a unit delay block after the
      | addition and before the signal split.
  note: Have to change size to 40 because
      |  LZC made for 40 bit number
  note: EFFECTIVELY shift_left(x_in,NShifts)
  x_in : Inport
  Bit Concat : hdlsllib/Logic and Bit Operations/Bit Concat  numInputs=2
      settings: SourceProductName=Simulink
  Bit Slice : hdlsllib/Logic and Bit Operations/Bit Slice  lidx=N_bits-1  ridx=0
      settings: SourceProductName=Simulink  SourceProductBaseCode=SL
  Bit Slice1 : hdlsllib/Logic and Bit Operations/Bit Slice  lidx=F_bits-1+d  ridx=F_bits-M_bits+d
      settings: SourceProductName=Simulink  SourceProductBaseCode=SL
  Bitwise Operator1 : simulink/Logic and Bit Operations/Bitwise Operator  logicop=NOT  UseBitMask=off  BitMask=bin2dec('11011001')  BitMaskRealWorld=Stored Integer
  Constant6 : Constant  Value=0  OutDataTypeStr=fixdt(0,9,0)  SampleTime=-1
  Data Type Conversion : DataTypeConversion  OutDataTypeStr=fixdt(0,40,F_bits+40-W_bits)
  Delay1 : Delay  DelayLength=1  InitialCondition=min_val
  Delay2 : Delay  DelayLength=1  InitialCondition=min_val
  LSL(N) : Subsystem
  MATLAB Function : MATLAB Function  TreatAsAtomicUnit=on
  Offset : Constant  Value=W_bits-1-F_bits-d  OutDataTypeStr=fixdt(0,6,0)  SampleTime=-1
  Remove Sign : DataTypeConversion  OutDataTypeStr=fixdt(0,W_bits,F_bits)
  Subtract : Sum  Inputs=+-  OutDataTypeStr=Inherit: Same as first input
  Switch1 : Switch  Criteria=u2 ~= 0
  Threshold Check : simulink/Logic and Bit Operations/Compare To Constant  relop=>  const=2^N_bits -1  OutDataTypeStr=boolean
  addr_r : Outport  VectorParamsAs1DForOutWhenUnconnected=off
  wires:
  x_in/1 -> Remove Sign/1, Data Type Conversion/1
  Bit Slice1/1 -> Bit Concat/2  "M"
  Bitwise Operator1/1 -> Bit Concat/1  "addr(5 downto 2)"
  MATLAB Function/1(lzc_count) -> Subtract/1
  Bit Concat/1 -> Switch1/3
  Offset/1 -> Subtract/2
  Bit Slice/1 -> Bitwise Operator1/1, LSL(N)/1(NShifts)  "NShifts"
  Delay2/1 -> LSL(N)/2(x_in)
  LSL(N)/1(x_shifted) -> Bit Slice1/1
  Data Type Conversion/1 -> MATLAB Function/1(x)
  Constant6/1 -> Switch1/1
  Switch1/1 -> addr_r/1
  Threshold Check/1 -> Switch1/2
  Remove Sign/1 -> Delay2/1
  Subtract/1 -> Delay1/1
  Delay1/1 -> Bit Slice/1, Threshold Check/1

== system DSP_FPGA_Accelerated_Toolbox/Programmable Look-Up Table/Low_LUT ==
  note: Initialized
  wr_din : Inport
  wr_addr : Inport  Port=2
  wr_en : Inport  Port=3  OutDataTypeStr=boolean
  rd_addr : Inport  Port=4
  Signal Specification : SignalSpecification  OutDataTypeStr=fixdt(0,ram_size,0)  Dimensions=1
  Signal Specification1 : SignalSpecification  OutDataTypeStr=fixdt(0,ram_size,0)  Dimensions=1
  convert : DataTypeConversion  OutDataTypeStr=uint16
  convert1 : DataTypeConversion  OutDataTypeStr=uint16
  ram : UnitDelay  InitialCondition=Table_Init  SampleTime=-1  HasFrameUpgradeWarning=on
  ram_data : UnitDelay  SampleTime=-1  HasFrameUpgradeWarning=on
  select : Selector  IndexMode=Zero-based  InputPortWidth=2^ram_size  IndexOptions=Index vector (port)  Indices=[1 3]  OutputSizes=1
  select1 : Selector  IndexMode=Zero-based  InputPortWidth=2^ram_size  IndexOptions=Index vector (port)  Indices=[1 3]  OutputSizes=1
  switch : Switch  Criteria=u2 ~= 0
  wr_addr_d : UnitDelay  SampleTime=-1  HasFrameUpgradeWarning=on
  wr_port : Assignment  IndexMode=Zero-based  IndexOptions=Index vector (port)  Indices=1  OutputSizes=[1 1]
  wr_dout : Outport  VectorParamsAs1DForOutWhenUnconnected=off
  rd_dout : Outport  Port=2  VectorParamsAs1DForOutWhenUnconnected=off
  wires:
  ram_data/1 -> rd_dout/1
  Signal Specification/1 -> convert/1
  wr_addr/1 -> Signal Specification/1
  wr_port/1 -> switch/1
  switch/1 -> ram/1
  ram/1 -> wr_port/1, select/1, select1/1, switch/3
  wr_din/1 -> wr_port/2
  wr_en/1 -> switch/2
  rd_addr/1 -> Signal Specification1/1
  select/1 -> ram_data/1
  convert/1 -> wr_port/3, wr_addr_d/1
  convert1/1 -> select/2
  select1/1 -> wr_dout/1
  wr_addr_d/1 -> select1/2
  Signal Specification1/1 -> convert1/1

== system DSP_FPGA_Accelerated_Toolbox/Programmable Look-Up Table, Linear Scale/LinAddressing ==
  note: z-1 here
      |    	|
      |    	|
      |   	v
  note: If input > highest expected input,
  note: If input < floor threshold input,
      | use the output corresponding to
      | the floor threshold input.
  note: Note: simulation version of this block has no latency.
      | But, in VHDL the inputs are registered, delaying the signal by 1.
      | If testing a simulation, simply attach a unit delay block after the
      | addition and before the signal split.
  note: Have to change size to 40 because
      |  LZC made for 40 bit number
  note: EFFECTIVELY shift_left(x_in,NShifts)
  x_in : Inport
  Bit Concat : hdlsllib/Logic and Bit Operations/Bit Concat  numInputs=2
      settings: SourceProductName=Simulink
  Bit Slice : hdlsllib/Logic and Bit Operations/Bit Slice  lidx=N_bits-1  ridx=0
      settings: SourceProductName=Simulink  SourceProductBaseCode=SL
  Bit Slice1 : hdlsllib/Logic and Bit Operations/Bit Slice  lidx=F_bits-1+d  ridx=F_bits-M_bits+d
      settings: SourceProductName=Simulink  SourceProductBaseCode=SL
  Bitwise Operator1 : simulink/Logic and Bit Operations/Bitwise Operator  logicop=NOT  UseBitMask=off  BitMask=bin2dec('11011001')  BitMaskRealWorld=Stored Integer
  Constant6 : Constant  Value=0  OutDataTypeStr=fixdt(0,9,0)  SampleTime=-1
  Data Type Conversion : DataTypeConversion  OutDataTypeStr=fixdt(0,40,F_bits+40-W_bits)
  Delay1 : Delay  DelayLength=1  InitialCondition=min_val
  Delay2 : Delay  DelayLength=1  InitialCondition=min_val
  LSL(N) : Subsystem
  MATLAB Function : MATLAB Function  TreatAsAtomicUnit=on
  Offset : Constant  Value=W_bits-1-F_bits-d  OutDataTypeStr=fixdt(0,6,0)  SampleTime=-1
  Remove Sign : DataTypeConversion  OutDataTypeStr=fixdt(0,W_bits,F_bits)
  Subtract : Sum  Inputs=+-  OutDataTypeStr=Inherit: Same as first input
  Switch1 : Switch  Criteria=u2 ~= 0
  Threshold Check : simulink/Logic and Bit Operations/Compare To Constant  relop=>  const=2^N_bits -1  OutDataTypeStr=boolean
  addr_r : Outport  VectorParamsAs1DForOutWhenUnconnected=off
  wires:
  x_in/1 -> Remove Sign/1, Data Type Conversion/1
  Bit Slice1/1 -> Bit Concat/2  "M"
  Bitwise Operator1/1 -> Bit Concat/1  "addr(5 downto 2)"
  MATLAB Function/1(lzc_count) -> Subtract/1
  Bit Concat/1 -> Switch1/3
  Offset/1 -> Subtract/2
  Bit Slice/1 -> Bitwise Operator1/1, LSL(N)/1(NShifts)  "NShifts"
  Delay2/1 -> LSL(N)/2(x_in)
  LSL(N)/1(x_shifted) -> Bit Slice1/1
  Data Type Conversion/1 -> MATLAB Function/1(x)
  Constant6/1 -> Switch1/1
  Switch1/1 -> addr_r/1
  Threshold Check/1 -> Switch1/2
  Remove Sign/1 -> Delay2/1
  Subtract/1 -> Delay1/1
  Delay1/1 -> Bit Slice/1, Threshold Check/1

== system DSP_FPGA_Accelerated_Toolbox/Programmable Look-Up Table, Linear Scale/Low_LUT ==
  note: Initialized
  wr_din : Inport
  wr_addr : Inport  Port=2
  wr_en : Inport  Port=3  OutDataTypeStr=boolean
  rd_addr : Inport  Port=4
  Signal Specification : SignalSpecification  OutDataTypeStr=fixdt(0,ram_size,0)  Dimensions=1
  Signal Specification1 : SignalSpecification  OutDataTypeStr=fixdt(0,ram_size,0)  Dimensions=1
  convert : DataTypeConversion  OutDataTypeStr=uint16
  convert1 : DataTypeConversion  OutDataTypeStr=uint16
  ram : UnitDelay  InitialCondition=Table_Init  SampleTime=-1  HasFrameUpgradeWarning=on
  ram_data : UnitDelay  SampleTime=-1  HasFrameUpgradeWarning=on
  select : Selector  IndexMode=Zero-based  InputPortWidth=2^ram_size  IndexOptions=Index vector (port)  Indices=[1 3]  OutputSizes=1
  select1 : Selector  IndexMode=Zero-based  InputPortWidth=2^ram_size  IndexOptions=Index vector (port)  Indices=[1 3]  OutputSizes=1
  switch : Switch  Criteria=u2 ~= 0
  wr_addr_d : UnitDelay  SampleTime=-1  HasFrameUpgradeWarning=on
  wr_port : Assignment  IndexMode=Zero-based  IndexOptions=Index vector (port)  Indices=1  OutputSizes=[1 1]
  wr_dout : Outport  VectorParamsAs1DForOutWhenUnconnected=off
  rd_dout : Outport  Port=2  VectorParamsAs1DForOutWhenUnconnected=off
  wires:
  ram_data/1 -> rd_dout/1
  Signal Specification/1 -> convert/1
  wr_addr/1 -> Signal Specification/1
  wr_port/1 -> switch/1
  switch/1 -> ram/1
  ram/1 -> wr_port/1, select/1, select1/1, switch/3
  wr_din/1 -> wr_port/2
  wr_en/1 -> switch/2
  rd_addr/1 -> Signal Specification1/1
  select/1 -> ram_data/1
  convert/1 -> wr_port/3, wr_addr_d/1
  convert1/1 -> select/2
  select1/1 -> wr_dout/1
  wr_addr_d/1 -> select1/2
  Signal Specification1/1 -> convert1/1
